simulink library "Generator_Lib"  (R2026a)
settings: Solver=ode45  EnableMultiTasking=on
undefined symbols (not defined in the file or in its folder): DiscIntNeverNeededParam, K, Lambda, radps2rpm, tau, WT_Params, x0
libraries: fl_lib x24, nesl_utility x16, ee_lib x14, simulink x1
(part 2 of 2)

== system Generator_Lib/Simple/Torque Sensor ==
  Ideal Torque Sensor : fl_lib/Mechanical/Mechanical Sensors/Ideal Torque Sensor
  PS-Simulink Converter : nesl_utility/PS-Simulink Converter  PhysicalDomain=network_engine_domain  SubClassName=ps_output  LeftPortType=input  RightPortType=output  PseudoPeriodic=off  Frequencies=[]  VectorFormat=1-D array  Unit=1  AffineConversion=off
  radps2rpm1 : Gain  Gain=1/500
  R : PMIOPort  Side=Left
  C : PMIOPort  Port=2  Side=Right
  tag scope: Gen_Torque_pu=global
  wires:
  radps2rpm1/1 -> [Gen_Torque_pu]  "Electromagnetic torque Te (pu)"
  PS-Simulink Converter/1 -> radps2rpm1/1
  connections:
  PS-Simulink Converter/LConn1 -- Ideal Torque Sensor/RConn2
  C/RConn1 -- Ideal Torque Sensor/RConn1
  R/RConn1 -- Ideal Torque Sensor/LConn1

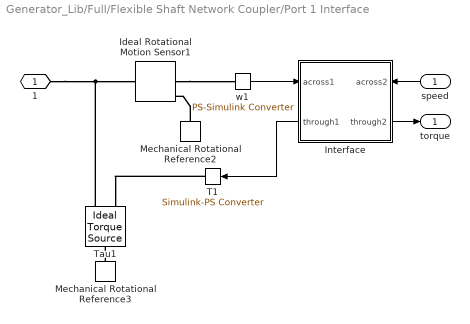
== system Generator_Lib/Full/Flexible Shaft Network Coupler/Port 1 Interface ==
  speed : Inport
  Ideal Rotational Motion Sensor1 : fl_lib/Mechanical/Mechanical Sensors/Ideal Rotational Motion Sensor  reference=foundation.enum.MeasurementReference.difference  acceleration_port=false  velocity_port=true  position_port=true  wrap_angle=simscape.enum.onoff.off  offset=0 rad
  Interface : Subsystem  Variant=on  VariantControlMode=label  VariantControl=Variant1  LabelModeActiveChoice=Continuous
      settings: PortSchema="{\"entries\":[{\"content\":{\"sides\":[{\"content\":{\"connectorIds\":[\"In1\",\"Out2\"]},\"type\":\"ConnectorPlacement.EquallySpacedRectSide\",\"uuid\":\"aa56821c-7799-44e3-b228-553c5b43a68d\"},{\"content\":{\"connectorIds\":[\"In2\",\"Out1\"],\"side\":\"RIGHT\"},\"type\":\"ConnectorPlacement.EquallySpacedRectSide\",\"uuid\":\"8658dee5-55e2-4f33-bdec-e6600ce27fc1\"},{\"content\":{\"connectorIds\":[],\"side\":\"TOP\"},\"type\":\"ConnectorPlacement.EquallySpacedRectSide\",\"uuid\":\"2effe9c6-8e61-4f0c-a39b-329d9ffc707d\"}]},\"type\":\"ConnectorPlacement.EquallySpacedConnector\",\"uuid\":\"c8fc8444-dfc7-49a5-9550-b957635f7d8f\"}],\"packageUris\":[\"http://schema.mathworks.com/mf0/Connector/R2020b\"],\"version\":\"1.0\"}"
  Mechanical Rotational Reference2 : fl_lib/Mechanical/Rotational Elements/Mechanical Rotational Reference
  Mechanical Rotational Reference3 : fl_lib/Mechanical/Rotational Elements/Mechanical Rotational Reference
  T1 : nesl_utility/Simulink-PS Converter  PhysicalDomain=network_engine_domain  SubClassName=ps_input  LeftPortType=input  RightPortType=output  PseudoPeriodic=off  Frequencies=[]  NoiseDistribution=none  NoiseParameters=[]  Unit=N*m  AffineConversion=off  FilteringAndDerivatives=zero  SimscapeFilterOrder=1  InputFilterTimeConstant=0.001  UdotUserProvided=1
  Tau1 : fl_lib/Mechanical/Mechanical Sources/Ideal Torque Source
  w1 : nesl_utility/PS-Simulink Converter  PhysicalDomain=network_engine_domain  SubClassName=ps_output  LeftPortType=input  RightPortType=output  PseudoPeriodic=off  Frequencies=[]  VectorFormat=1-D array  Unit=rad/s  AffineConversion=off
  1 : PMIOPort  Side=Left
  torque : Outport
  wires:
  speed/1 -> Interface/2(across2)
  Interface/2(through1) -> T1/1
  w1/1 -> Interface/1(across1)
  Interface/1(through2) -> torque/1
  connections:
  1/RConn1 -- Ideal Rotational Motion Sensor1/LConn1 -- Tau1/RConn2
  Mechanical Rotational Reference2/LConn1 -- Ideal Rotational Motion Sensor1/RConn1
  Ideal Rotational Motion Sensor1/RConn2 -- w1/LConn1
  Mechanical Rotational Reference3/LConn1 -- Tau1/LConn1
  T1/RConn1 -- Tau1/RConn1

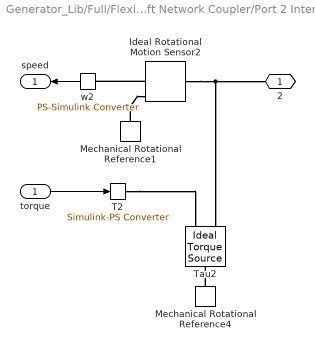
== system Generator_Lib/Full/Flexible Shaft Network Coupler/Port 2 Interface ==
  torque : Inport
  Ideal Rotational Motion Sensor2 : fl_lib/Mechanical/Mechanical Sensors/Ideal Rotational Motion Sensor  reference=foundation.enum.MeasurementReference.difference  acceleration_port=false  velocity_port=true  position_port=true  wrap_angle=simscape.enum.onoff.off  offset=0 rad
  Mechanical Rotational Reference1 : fl_lib/Mechanical/Rotational Elements/Mechanical Rotational Reference
  Mechanical Rotational Reference4 : fl_lib/Mechanical/Rotational Elements/Mechanical Rotational Reference
  T2 : nesl_utility/Simulink-PS Converter  PhysicalDomain=network_engine_domain  SubClassName=ps_input  LeftPortType=input  RightPortType=output  PseudoPeriodic=off  Frequencies=[]  NoiseDistribution=none  NoiseParameters=[]  Unit=N*m  AffineConversion=off  FilteringAndDerivatives=zero  SimscapeFilterOrder=1  InputFilterTimeConstant=0.001  UdotUserProvided=1
  Tau2 : fl_lib/Mechanical/Mechanical Sources/Ideal Torque Source
  w2 : nesl_utility/PS-Simulink Converter  PhysicalDomain=network_engine_domain  SubClassName=ps_output  LeftPortType=input  RightPortType=output  PseudoPeriodic=off  Frequencies=[]  VectorFormat=1-D array  Unit=rad/s  AffineConversion=off
  2 : PMIOPort  Side=Right
  speed : Outport
  wires:
  torque/1 -> T2/1
  w2/1 -> speed/1
  connections:
  T2/RConn1 -- Tau2/RConn1
  Mechanical Rotational Reference1/LConn1 -- Ideal Rotational Motion Sensor2/RConn1
  Ideal Rotational Motion Sensor2/RConn2 -- w2/LConn1
  Ideal Rotational Motion Sensor2/LConn1 -- 2/RConn1 -- Tau2/RConn2
  Mechanical Rotational Reference4/LConn1 -- Tau2/LConn1

== system Generator_Lib/Full/Measurements/Filter ==
  In : Inport
  Gain : Gain  Gain=1/b
  Integrator : Integrator  InitialCondition=x_initial
  Sum : Sum  Inputs=|+-  InputSameDT=on  SaturateOnIntegerOverflow=on  OutDataTypeStr=Inherit: Same as first input
  Out : Outport  VectorParamsAs1DForOutWhenUnconnected=off
  wires:
  Gain/1 -> Out/1, Sum/2
  Integrator/1 -> Gain/1
  In/1 -> Sum/1
  Sum/1 -> Integrator/1

== system Generator_Lib/Full/Flexible Shaft Network Coupler/Port 1 Interface/Interface ==
  across1 : Inport
  across2 : Inport  Port=2
  Continuous : Subsystem  VariantControl=Continuous
  Discrete : Subsystem  VariantControl=Discrete
  through2 : Outport
  through1 : Outport  Port=2

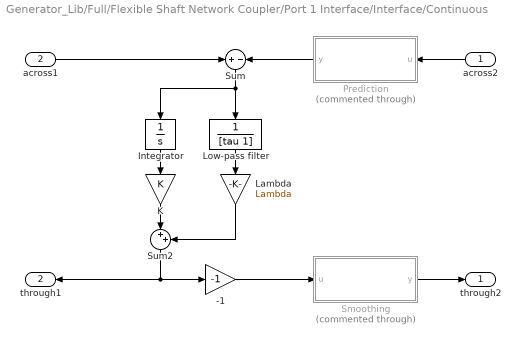
== system Generator_Lib/Full/Flexible Shaft Network Coupler/Port 1 Interface/Interface/Continuous ==
  across2 : Inport
  across1 : Inport  Port=2
  -1 : Gain  Gain=-1  SaturateOnIntegerOverflow=on  OutDataTypeStr=Inherit: Same as input  ParamDataTypeStr=Inherit: Same as input
  Integrator : Integrator  InitialCondition=x0
  K : Gain  Gain=K  SaturateOnIntegerOverflow=on  OutDataTypeStr=Inherit: Same as input  ParamDataTypeStr=Inherit: Same as input
  Lambda : Gain  Gain=Lambda  SaturateOnIntegerOverflow=on  OutDataTypeStr=Inherit: Same as input  ParamDataTypeStr=Inherit: Same as input
  Low-pass filter : TransferFcn  Numerator=1  Denominator=[tau 1]
  Prediction : Subsystem  Commented=through  mask(Prediction (discrete->continuous)){h2=h2}
      mask prompts: h2 "physmod:simscape:couplers:SimscapeNetworkCouplersLib:PortUDiscreteSampleTimes_MP"
      mask help: physmod:simscape:couplers:SimscapeNetworkCouplersLib:Predictiondiscretecontinuous_MD
      mask DialogControl h2 Prompt: Port u discrete sample time (s)
  Smoothing : Subsystem  Commented=through  mask(Smoothing (continuous->discrete)){tsSmoothing=tsSmoothing, smoothing0=-through0}
      mask prompts: tsSmoothing "physmod:simscape:couplers:SimscapeNetworkCouplersLib:SmoothingTimeConstants_MP"; smoothing0 "physmod:simscape:couplers:SimscapeNetworkCouplersLib:InitialOutput_MP"
      mask help: physmod:simscape:couplers:SimscapeNetworkCouplersLib:Smoothingcontinuousdiscrete_MD
      mask DialogControl tsSmoothing Prompt: Smoothing time constant (s)
      mask DialogControl smoothing0 Prompt: Initial output
  Sum : Sum  Inputs=+-  InputSameDT=on  SaturateOnIntegerOverflow=on  OutDataTypeStr=Inherit: Same as first input
  Sum2 : Sum  Inputs=|++
  through2 : Outport
  through1 : Outport  Port=2
  wires:
  K/1 -> Sum2/1
  Sum2/1 -> through1/1, -1/1
  across2/1 -> Prediction/1(u)
  Low-pass filter/1 -> Lambda/1
  Integrator/1 -> K/1
  Sum/1 -> Integrator/1, Low-pass filter/1
  across1/1 -> Sum/1
  Lambda/1 -> Sum2/2
  Prediction/1(y) -> Sum/2
  Smoothing/1(y) -> through2/1
  -1/1 -> Smoothing/1(u)

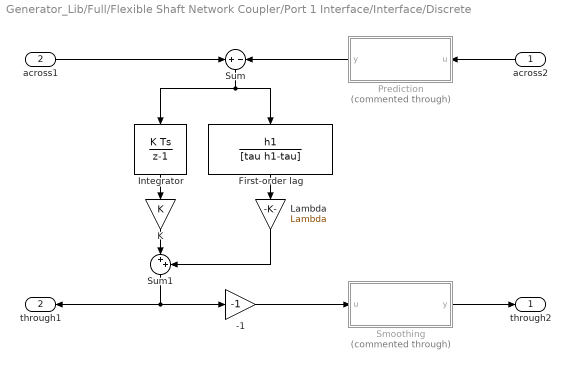
== system Generator_Lib/Full/Flexible Shaft Network Coupler/Port 1 Interface/Interface/Discrete ==
  across2 : Inport
  across1 : Inport  Port=2
  -1 : Gain  Gain=-1  SaturateOnIntegerOverflow=on  OutDataTypeStr=Inherit: Same as input  ParamDataTypeStr=Inherit: Same as input
  First-order lag : DiscreteTransferFcn  Numerator=h1  Denominator=[tau h1-tau]  SampleTime=h1
  Integrator : DiscreteIntegrator  InitialCondition=x0  SampleTime=h1  ICPrevOutput=DiscIntNeverNeededParam  ICPrevScaledInput=DiscIntNeverNeededParam
  K : Gain  Gain=K  SaturateOnIntegerOverflow=on  OutDataTypeStr=Inherit: Same as input  ParamDataTypeStr=Inherit: Same as input
  Lambda : Gain  Gain=Lambda  SaturateOnIntegerOverflow=on  OutDataTypeStr=Inherit: Same as input  ParamDataTypeStr=Inherit: Same as input
  Prediction : Subsystem  Commented=through  mask(Prediction (slow->fast)){h2=h2, h1=h1}
      mask prompts: h2 "physmod:simscape:couplers:SimscapeNetworkCouplersLib:PortUDiscreteSampleTimes_MP"; h1 "physmod:simscape:couplers:SimscapeNetworkCouplersLib:PortYDiscreteSampleTimes_MP"
      mask help: physmod:simscape:couplers:SimscapeNetworkCouplersLib:Predictionslowfast_MD
      mask DialogControl h2 Prompt: Port u discrete sample time (s)
      mask DialogControl h1 Prompt: Port y discrete sample time (s)
  Smoothing : Subsystem  Commented=through  mask(Smoothing (fast->slow)){nSmooth=nSmooth, h1=h1, smoothing0=-through0}
      mask prompts: nSmooth "physmod:simscape:couplers:SimscapeNetworkCouplersLib:NumberOfSamplesOverWhichToSmooth_MP"; h1 "physmod:simscape:couplers:SimscapeNetworkCouplersLib:PortUDiscreteSampleTimes_MP"; smoothing0 "physmod:simscape:couplers:SimscapeNetworkCouplersLib:InitialOutput_MP"
      mask help: physmod:simscape:couplers:SimscapeNetworkCouplersLib:Smoothingfastslow_MD
      mask DialogControl nSmooth Prompt: Number of samples over which to smooth
      mask DialogControl h1 Prompt: Port u discrete sample time (s)
      mask DialogControl smoothing0 Prompt: Initial output
  Sum : Sum  Inputs=+-  InputSameDT=on  SaturateOnIntegerOverflow=on  OutDataTypeStr=Inherit: Same as first input
  Sum1 : Sum  Inputs=|++
  through2 : Outport
  through1 : Outport  Port=2
  wires:
  First-order lag/1 -> Lambda/1
  Integrator/1 -> K/1
  K/1 -> Sum1/1
  across1/1 -> Sum/1
  Sum/1 -> Integrator/1, First-order lag/1
  across2/1 -> Prediction/1(u)
  Sum1/1 -> through1/1, -1/1
  Lambda/1 -> Sum1/2
  Prediction/1(y) -> Sum/2
  Smoothing/1(y) -> through2/1
  -1/1 -> Smoothing/1(u)

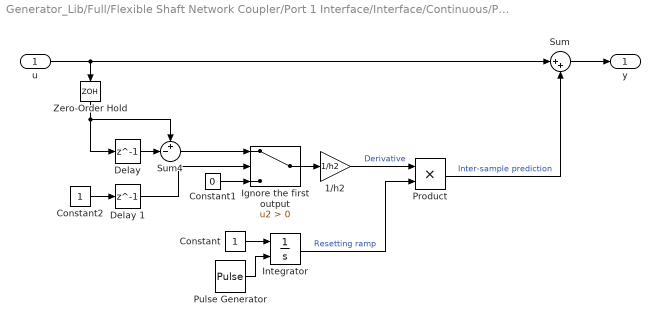
== system Generator_Lib/Full/Flexible Shaft Network Coupler/Port 1 Interface/Interface/Continuous/Prediction ==
  u : Inport
  1/h2 : Gain  Gain=1/h2
  Constant : Constant  SampleTime=h2
  Constant1 : Constant  Value=0  SampleTime=h2
  Constant2 : Constant  SampleTime=h2
  "Delay " : Delay  DelayLength=1  SampleTime=h2
  Delay 1 : Delay  DelayLength=1  SampleTime=h2
  Ignore the first output : Switch  Criteria=u2 > Threshold  SaturateOnIntegerOverflow=off  InputSameDT=off
  Integrator : Integrator  ExternalReset=either  LimitOutput=on  UpperSaturationLimit=1  LowerSaturationLimit=0
  Product : Product
  Pulse Generator : DiscretePulseGenerator  SampleTime=h2
  Sum : Sum  Inputs=|++
  Sum4 : Sum  Inputs=+-|
  Zero-Order Hold : ZeroOrderHold  SampleTime=h2
  y : Outport
  wires:
  Product/1 -> Sum/2  "Inter-sample prediction"
  Zero-Order Hold/1 -> Sum4/1, "Delay "/1
  u/1 -> Sum/1, Zero-Order Hold/1
  "Delay "/1 -> Sum4/2
  1/h2/1 -> Product/1  "Derivative"
  Sum/1 -> y/1
  Integrator/1 -> Product/2  "Resetting ramp"
  Constant/1 -> Integrator/1
  Pulse Generator/1 -> Integrator/2
  Ignore the first output/1 -> 1/h2/1
  Sum4/1 -> Ignore the first output/1
  Constant1/1 -> Ignore the first output/3
  Delay 1/1 -> Ignore the first output/2
  Constant2/1 -> Delay 1/1

== system Generator_Lib/Full/Flexible Shaft Network Coupler/Port 1 Interface/Interface/Continuous/Smoothing ==
  u : Inport
  Gain : Gain  Gain=1/tsSmoothing
  Integrator : Integrator  InitialCondition=smoothing0
  Sum : Sum  Inputs=|+-
  y : Outport
  wires:
  u/1 -> Sum/1
  Integrator/1 -> Sum/2, y/1
  Gain/1 -> Integrator/1
  Sum/1 -> Gain/1

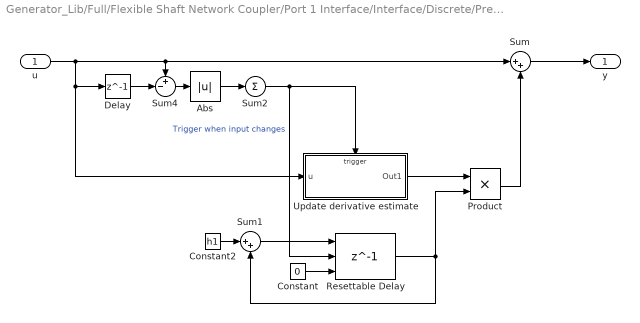
== system Generator_Lib/Full/Flexible Shaft Network Coupler/Port 1 Interface/Interface/Discrete/Prediction ==
  u : Inport
  Abs : Abs  SaturateOnIntegerOverflow=off
  Constant : Constant  Value=0  SampleTime=h1
  Constant2 : Constant  Value=h1  SampleTime=h1
  "Delay " : Delay  DelayLength=1  SampleTime=h1
  Product : Product
  Resettable Delay : Delay  DelayLength=1  InitialConditionSource=Input port  ExternalReset=Rising  SampleTime=h1
      settings: InputPortMap=u0,r5,p4
  Sum : Sum  Inputs=|++
  Sum1 : Sum  Inputs=|++
  Sum2 : Sum  Inputs=+
  Sum4 : Sum  Inputs=+-|
  Update derivative estimate : Subsystem  TreatAsAtomicUnit=on
  y : Outport
  wires:
  Abs/1 -> Sum2/1
  Sum2/1 -> Resettable Delay/2, Update derivative estimate/Trigger  "Trigger when input changes"
  Sum1/1 -> Resettable Delay/1
  Sum/1 -> y/1
  "Delay "/1 -> Sum4/2
  Product/1 -> Sum/2
  Update derivative estimate/1(Out1) -> Product/1
  u/1 -> Update derivative estimate/1(u), "Delay "/1, Sum/1, Sum4/1
  Sum4/1 -> Abs/1
  Resettable Delay/1 -> Product/2, Sum1/2
  Constant2/1 -> Sum1/1
  Constant/1 -> Resettable Delay/3

== system Generator_Lib/Full/Flexible Shaft Network Coupler/Port 1 Interface/Interface/Discrete/Smoothing ==
  u : Inport
  Gain : Gain  Gain=1/nSmooth
  Sum of Elements : Sum  Inputs=+
  Tapped Delay : simulink/Discrete/Tapped Delay  vinit=smoothing0  samptime=h1  NumDelays=nSmooth  DelayOrder=Oldest  includeCurrent=off
  y : Outport
  wires:
  Gain/1 -> y/1
  Sum of Elements/1 -> Gain/1
  Tapped Delay/1 -> Sum of Elements/1
  u/1 -> Tapped Delay/1

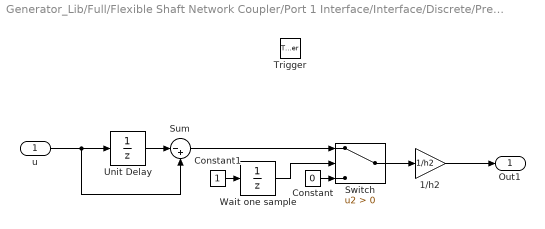
== system Generator_Lib/Full/Flexible Shaft Network Coupler/Port 1 Interface/Interface/Discrete/Prediction/Update derivative estimate ==
  u : Inport
  Trigger : TriggerPort  VariantControl=(inherit)
  1/h2 : Gain  Gain=1/h2
  Constant : Constant  Value=0  SampleTime=-1
  Constant1 : Constant  SampleTime=-1
  Sum : Sum  Inputs=|-+
  Switch : Switch  Criteria=u2 > Threshold  SaturateOnIntegerOverflow=off  InputSameDT=off
  Unit Delay : UnitDelay  SampleTime=-1
  Wait one sample : UnitDelay  SampleTime=-1
  Out1 : Outport
  wires:
  Unit Delay/1 -> Sum/1
  u/1 -> Unit Delay/1, Sum/2
  1/h2/1 -> Out1/1
  Switch/1 -> 1/h2/1
  Sum/1 -> Switch/1
  Constant/1 -> Switch/3
  Wait one sample/1 -> Switch/2
  Constant1/1 -> Wait one sample/1
